simulink library "M160_lib"  (Simulink 7.8)
settings: Solver=FixedStepDiscrete  StartTime=0.0  StopTime=10.0  RelTol=1e-3
PreLoadFcn:
  | update_path
undefined symbols (not defined in the file): Afr_atCool2facLambdaReqCorr_CUR_x, Afr_atCool2facLambdaReqCorr_CUR_y, Afr_atMani2facLambdaReqCorr_CUR_x, Afr_atMani2facLambdaReqCorr_CUR_y, Afr_facLambdaReqMan, Afr_facRatioMan, Afr_facStoich, Afr_flgLambdaReqOverride, Afr_flgRatioOverride, Afr_rpmEngSpdfacRelAir2facLambdaReqBase_MAP_x, Afr_rpmEngSpdfacRelAir2facLambdaReqBase_MAP_y, Afr_rpmEngSpdfacRelAir2facLambdaReqBase_MAP_z, Ais_flgAirInjReacPumpOverride, Ais_stAirInjReacPumpMan, Amc_flgAirMassFlowOverride, Amc_uSens2AirMassFlow_CUR_x, Amc_uSens2AirMassFlow_CUR_y, Amc_uSensMaxValid, Amc_uSensMinValid, Amf_facRelAirMan, Amf_flgAirMassPerStrOverride, Amf_flgRelAirOverride, Amf_flgSwitch2AirMassFlowMeter, Amf_mAirPerStrMan, Amf_pManiEngSpd2facRelAirCorr_MAP_x, Amf_pManiEngSpd2facRelAirCorr_MAP_y, Amf_pManiEngSpd2facRelAirCorr_MAP_z, Amf_rpmEngSpd2facTempCorr_CUR_x, Amf_rpmEngSpd2facTempCorr_CUR_y, Amf_shcSpecGasConst_C, Amf_volEngDisp_C, Apv_facAirPumpRateMan, Apv_factor, Apv_flgAirPumpRateOverride, Apv_tiPeriod_C, Bvc_rVoltDivHigh, Bvc_rVoltDivLow, Bvc_uBattMax, Bvc_uBattMin, CDRV_E_OK_, Cov_facChOverVlvRateMan, Cov_factor, Cov_flgChOverVlvRateOverride, Cov_tiPeriod_C, Cpc_atManiTmp2facPresCorr_CUR_x, Cpc_atManiTmp2facPresCorr_CUR_y, Cpc_flgPChargeOverride, Cpc_uSens2pManiBase_CUR_x, Cpc_uSens2pManiBase_CUR_y, Ctc_rPullUp_C, Ctc_rSens2atCool_CUR_x, Ctc_rSens2atCool_CUR_y, Ctc_uSensMaxValid, Ctc_uSensMinValid, Ctc_uSupply, Doh_OutputDiagnosisOverride, dummy_facAirPumpRateReq, dummy_facChOverVlvRateReq, dummy_flgInterCoolerOverride, dummy_flgKl50Override ... (+243)
libraries: simulink x36, ehooks_lib x3
(part 5 of 8)

== system M160_lib/Actuators/Ivc/Ivc ==
  Opm_idxMode : Inport
  Itc_flgInjCutoff : Inport  Port=2
  Itc_tiInj : Inport  Port=3
  Itc_tiBattDelay : Inport  Port=4
  function : TriggerPort  TriggerType=function-call
  Constant1 : Constant  Value=Ivc_flgInjCutoffOverride
  Constant10 : Constant  Value=Ivc_flgEndOfStartCond
  Constant11 : Constant  Value=Ivc_tiMinThresDeltaEffInjPeriod
  Constant{6,12..15} (5 alike) : Constant  Value=0  OutMin=-72  OutMax=78  OutDataTypeStr=single
  Constant16 : Constant  Value=255  OutDataTypeStr=single
  Constant17 : Constant  Value=0  OutDataTypeStr=single
  Constant18 : Constant  Value=Ivc_tiBattDelayMan
  Constant19 : Constant  Value=Ivc_flgBattDelayOverride
  Constant2 : Constant  Value=Ivc_flgInjCutoff
  Constant20 : Constant  Value=Ivc_degInjAbort
  Constant21 : Constant  Value=Ivc_weea0
  Constant22 : Constant  Value=Ivc_weea1
  Constant23 : Constant  Value=Ivc_weea2
  Constant24 : Constant  Value=Ivc_degOffsetInjEndSimultanInj
  Constant25 : Constant  Value=Ivc_degIntakeClose
  Constant3 : Constant  Value=CDRV_E_OK_
  Constant4 : Constant  Value=Ivc_flgInjTimeOverride
  Constant5 : Constant  Value=Normal
  Constant7 : Constant  Value=Ivc_tiInjMan
  Constant8 : Constant  Value=Ivc_tiInjEff
  Constant9 : Constant  Value=Ivc_flgPostInjCond
  Demux : Demux  Outputs=8
  Demux2 : Demux  Outputs=3
  G1_InjVlvPFI_SetParam : Subsystem  AncestorBlock=ehooks_medc17flex_G1_lib/Library Blocks/INJ/PFI/G1_InjVlvPFI_SetParam  LoadFcn=ehooks_medc17flex_devlib_io_block('load');  InitFcn=ehooks_medc17flex_devlib_io_block('init');  StartFcn=ehooks_medc17flex_devlib_io_block('start');  StopFcn=ehooks_medc17flex_devlib_io_block('stop');  ClipboardFcn=ehooks_medc17flex_devlib_io_block('clipboard', 0); % Second argument just needed to indicate null block. See callback handler.  mask{ChannelName=IGNORED}
      mask prompts: ChannelName "PlaceHolder_IGNORED"
      mask init:
      | ehooks_medc17flex_devlib_io_block('mask_init');
      settings: CopyFcn=ehooks_medc17flex_devlib_io_block('copy');  DeleteFcn=ehooks_medc17flex_devlib_io_block('delete');  UndoDeleteFcn=ehooks_medc17flex_devlib_io_block('undo_delete');  ModelCloseFcn=ehooks_medc17flex_devlib_io_block('model_close');  PreSaveFcn=ehooks_medc17flex_devlib_io_block('pre_save');  PostSaveFcn=ehooks_medc17flex_devlib_io_block('post_save');  NameChangeFcn=ehooks_medc17flex_devlib_io_block('name_change');  DestroyFcn=ehooks_medc17flex_devlib_io_block('destroy', 0); % Second argument just needed to indicate null block. See callback handler.  OpenFcn=ehooks_medc17flex_devlib_io_block('open');  CloseFcn=ehooks_medc17flex_devlib_io_block('close');  ParentCloseFcn=ehooks_medc17flex_devlib_io_block('parent_close');  MoveFcn=ehooks_medc17flex_devlib_io_block('move');
      mask StyleString: popup(IGNORED)
      mask Display: image(imread('InjVlvPfi.jpg'))
  Logical Operator3 : Logic  Operator=OR  AllPortsSameDT=off  OutDataTypeStr=boolean
  Relational Operator : RelationalOperator  Operator=~=  OutDataTypeStr=boolean
  Relational Operator1 : RelationalOperator  Operator=~=  OutDataTypeStr=boolean
  Switch{1..4} (4 alike) : Switch  Threshold=1
  Vector Concatenate : Concatenate  NumInputs=8  Mode=Vector
  Vector Concatenate1 : Concatenate  NumInputs=3  Mode=Vector
  Ivc_flgError : Outport
  wires:
  Switch2/1 -> Vector Concatenate/1, Vector Concatenate/2, Vector Concatenate/3
  Constant15/1 -> Vector Concatenate/8
  Constant14/1 -> Vector Concatenate/7
  Constant13/1 -> Vector Concatenate/6
  Constant12/1 -> Vector Concatenate/5
  Constant6/1 -> Vector Concatenate/4
  Vector Concatenate/1 -> Demux/1  "Ivc_tiInjEffCylInd_Arr"
  Constant8/1 -> G1_InjVlvPFI_SetParam/1(te_i)
  Switch1/1 -> Logical Operator3/2
  Relational Operator/1 -> Logical Operator3/1
  Constant7/1 -> Switch2/1
  Constant4/1 -> Switch2/2
  Itc_tiInj/1 -> Switch2/3
  Constant3/1 -> Relational Operator1/2
  Relational Operator1/1 -> Ivc_flgError/1
  G1_InjVlvPFI_SetParam/1(Cdrv_Error) -> Relational Operator1/1  "Ivc_idxPfiCdrvInterfaceError"
  Constant5/1 -> Relational Operator/2
  Opm_idxMode/1 -> Relational Operator/1
  Itc_flgInjCutoff/1 -> Switch1/3
  Constant2/1 -> Switch1/1
  Constant1/1 -> Switch1/2
  Logical Operator3/1 -> Switch3/2
  Constant16/1 -> Switch3/1
  Constant17/1 -> Switch3/3
  Switch3/1 -> [Ivc_stCutoffPattern_local]  "Ivc_stCutoffPattern"
  Constant18/1 -> Switch4/1
  Constant19/1 -> Switch4/2
  Itc_tiBattDelay/1 -> Switch4/3
  Vector Concatenate1/1 -> Demux2/1  "Ivc_degInjEnd"
  Constant21/1 -> Vector Concatenate1/1
  Constant22/1 -> Vector Concatenate1/2
  Constant23/1 -> Vector Concatenate1/3
  Switch4/1 -> G1_InjVlvPFI_SetParam/11(tvub_w)  "Ivc_tiBattDelay"
  Constant11/1 -> G1_InjVlvPFI_SetParam/10(dtemnkt_w)
  Demux/1 -> G1_InjVlvPFI_SetParam/2(tez_i1)
  Demux/2 -> G1_InjVlvPFI_SetParam/3(tez_i2)
  Demux/3 -> G1_InjVlvPFI_SetParam/4(tez_i3)
  Demux/4 -> G1_InjVlvPFI_SetParam/5(tez_i4)
  Demux/5 -> G1_InjVlvPFI_SetParam/6(tez_i5)
  Demux/6 -> G1_InjVlvPFI_SetParam/7(tez_i6)
  Demux/7 -> G1_InjVlvPFI_SetParam/8(tez_i7)
  Demux/8 -> G1_InjVlvPFI_SetParam/9(tez_i8)
  Constant9/1 -> G1_InjVlvPFI_SetParam/12(B_nsp)
  Constant10/1 -> G1_InjVlvPFI_SetParam/13(B_stendes)
  [Ivc_stCutoffPattern_local] -> G1_InjVlvPFI_SetParam/14(evz_austot)
  Constant20/1 -> G1_InjVlvPFI_SetParam/15(wea)
  Demux2/1 -> G1_InjVlvPFI_SetParam/16(weea_1)
  Demux2/2 -> G1_InjVlvPFI_SetParam/17(weea_2)
  Demux2/3 -> G1_InjVlvPFI_SetParam/18(weea_3)
  Constant24/1 -> G1_InjVlvPFI_SetParam/19(weestim)
  Constant25/1 -> G1_InjVlvPFI_SetParam/20(wes)

== system M160_lib/Actuators/Ivc/Ivc_Diag ==
  function : TriggerPort  TriggerType=function-call
  Constant3 : Constant  Value=CDRV_E_OK_
  Constant8 : Constant  Value=Ivc_flgDiagEntryCondFulfilled
  Constant9 : Constant  Value=Ivc_flgOverrunCutoff
  G1_Inj_Set_DEVE_forPFI : Subsystem  AncestorBlock=ehooks_medc17flex_G1_lib/Library Blocks/INJ/PFI/G1_Inj_Set_DEVE_forPFI  LoadFcn=ehooks_medc17flex_devlib_io_block('load');  InitFcn=ehooks_medc17flex_devlib_io_block('init');  StartFcn=ehooks_medc17flex_devlib_io_block('start');  StopFcn=ehooks_medc17flex_devlib_io_block('stop');  ClipboardFcn=ehooks_medc17flex_devlib_io_block('clipboard', 0); % Second argument just needed to indicate null block. See callback handler.  mask{ChannelName=IGNORED}
      mask prompts: ChannelName "PlaceHolder_IGNORED"
      mask help: InjVlvDeve
      mask init:
      | ehooks_medc17flex_devlib_io_block('mask_init');
      settings: CopyFcn=ehooks_medc17flex_devlib_io_block('copy');  DeleteFcn=ehooks_medc17flex_devlib_io_block('delete');  UndoDeleteFcn=ehooks_medc17flex_devlib_io_block('undo_delete');  ModelCloseFcn=ehooks_medc17flex_devlib_io_block('model_close');  PreSaveFcn=ehooks_medc17flex_devlib_io_block('pre_save');  PostSaveFcn=ehooks_medc17flex_devlib_io_block('post_save');  NameChangeFcn=ehooks_medc17flex_devlib_io_block('name_change');  DestroyFcn=ehooks_medc17flex_devlib_io_block('destroy', 0); % Second argument just needed to indicate null block. See callback handler.  OpenFcn=ehooks_medc17flex_devlib_io_block('open');  CloseFcn=ehooks_medc17flex_devlib_io_block('close');  ParentCloseFcn=ehooks_medc17flex_devlib_io_block('parent_close');  MoveFcn=ehooks_medc17flex_devlib_io_block('move');
      mask StyleString: popup(IGNORED)
      mask Display: image(imread('InjVlvPfi.jpg'))
  Relational Operator1 : RelationalOperator  Operator=~=  OutDataTypeStr=boolean
  Ivc_flgError : Outport
  wires:
  G1_Inj_Set_DEVE_forPFI/1(Cdrv_Error) -> Relational Operator1/1  "Ivc_idxDeveCdrvInterfaceError"
  Relational Operator1/1 -> Ivc_flgError/1
  Constant3/1 -> Relational Operator1/2
  Constant9/1 -> G1_Inj_Set_DEVE_forPFI/2(B_sa)
  Constant8/1 -> G1_Inj_Set_DEVE_forPFI/1(B_desee)

== system M160_lib/Actuators/Ivc/Ivc_Error ==
  Ivc : Inport
  Ivc_Diag : Inport  Port=2
  function : TriggerPort  TriggerType=function-call
  Logical Operator3 : Logic  Operator=OR  AllPortsSameDT=off  OutDataTypeStr=boolean
  Ivc_flgError : Outport
  wires:
  Logical Operator3/1 -> Ivc_flgError/1  "Ivc_flgError"
  Ivc/1 -> Logical Operator3/1
  Ivc_Diag/1 -> Logical Operator3/2

== system M160_lib/Actuators/Mrs/G1_DigOut_Ctrl ==
  state : Inport
  DTC_DigOut_ctrl : DataTypeConversion  OutDataTypeStr=uint8  RndMeth=Nearest
  DTC_Out1 : DataTypeConversion  OutDataTypeStr=boolean
  FlexECU_DevLib_FcnAPI_Wrapper_SFcn : S-Function  FunctionName=ehooks_medc17flex_devlib_basic_io_fcncall  Parameters=NoInputPorts, NoOutputPorts, InputPortDataTypes, OutputPortDataTypes, CFunctionArgTypes, CFunctionName, ChannelName  EnableBusSupport=off  mask{NoInputPorts=1, NoOutputPorts=1, InputPortDataTypes=uint8, OutputPortDataTypes=uint8, CFunctionArgTypes=ret,val, CFunctionName=DevLib_Dio_Set, ChannelName=O_S_MRLY}
      mask prompts: NoInputPorts "Number of input ports"; NoOutputPorts "Number of output ports"; InputPortDataTypes "Input port data types"; OutputPortDataTypes "Output port data types"; CFunctionArgTypes "C function argument types"; CFunctionName "C function name"; ChannelName "Channel (pin) name"
      mask Display: disp('EHOOKS FlexECU\nDevLib Wrapper\nS-Function')
  status : Outport
  wires:
  DTC_DigOut_ctrl/1 -> FlexECU_DevLib_FcnAPI_Wrapper_SFcn/1
  state/1 -> DTC_DigOut_ctrl/1
  FlexECU_DevLib_FcnAPI_Wrapper_SFcn/1 -> DTC_Out1/1
  DTC_Out1/1 -> status/1

== system M160_lib/Actuators/Mrs/G1_DigOut_GetError ==
  DTC_DigOut_GetError : DataTypeConversion  OutDataTypeStr=single
  FlexECU_DevLib_FcnAPI_Wrapper_SFcn : S-Function  FunctionName=ehooks_medc17flex_devlib_basic_io_fcncall  Parameters=NoInputPorts, NoOutputPorts, InputPortDataTypes, OutputPortDataTypes, CFunctionArgTypes, CFunctionName, ChannelName  EnableBusSupport=off  mask{NoInputPorts=0, NoOutputPorts=1, InputPortDataTypes=, OutputPortDataTypes=uint8, CFunctionArgTypes=ret, CFunctionName=DevLib_DioSet_GetError, ChannelName=O_S_MRLY}
      mask prompts: NoInputPorts "Number of input ports"; NoOutputPorts "Number of output ports"; InputPortDataTypes "Input port data types"; OutputPortDataTypes "Output port data types"; CFunctionArgTypes "C function argument types"; CFunctionName "C function name"; ChannelName "Channel (pin) name"
      mask Display: disp('EHOOKS FlexECU\nDevLib Wrapper\nS-Function')
  status : Outport
  wires:
  DTC_DigOut_GetError/1 -> status/1
  FlexECU_DevLib_FcnAPI_Wrapper_SFcn/1 -> DTC_DigOut_GetError/1

== system M160_lib/Actuators/Str/G1_DigOut_Ctrl ==
  state : Inport
  DTC_DigOut_ctrl : DataTypeConversion  OutDataTypeStr=uint8  RndMeth=Nearest
  DTC_Out1 : DataTypeConversion  OutDataTypeStr=boolean
  FlexECU_DevLib_FcnAPI_Wrapper_SFcn : S-Function  FunctionName=ehooks_medc17flex_devlib_basic_io_fcncall  Parameters=NoInputPorts, NoOutputPorts, InputPortDataTypes, OutputPortDataTypes, CFunctionArgTypes, CFunctionName, ChannelName  EnableBusSupport=off  mask{NoInputPorts=1, NoOutputPorts=1, InputPortDataTypes=uint8, OutputPortDataTypes=uint8, CFunctionArgTypes=ret,val, CFunctionName=DevLib_Dio_Set, ChannelName=O_S_RL34}
      mask prompts: NoInputPorts "Number of input ports"; NoOutputPorts "Number of output ports"; InputPortDataTypes "Input port data types"; OutputPortDataTypes "Output port data types"; CFunctionArgTypes "C function argument types"; CFunctionName "C function name"; ChannelName "Channel (pin) name"
      mask Display: disp('EHOOKS FlexECU\nDevLib Wrapper\nS-Function')
  status : Outport
  wires:
  DTC_DigOut_ctrl/1 -> FlexECU_DevLib_FcnAPI_Wrapper_SFcn/1
  state/1 -> DTC_DigOut_ctrl/1
  FlexECU_DevLib_FcnAPI_Wrapper_SFcn/1 -> DTC_Out1/1
  DTC_Out1/1 -> status/1

== system M160_lib/Actuators/Str/G1_DigOut_GetError ==
  DTC_DigOut_GetError : DataTypeConversion  OutDataTypeStr=single
  FlexECU_DevLib_FcnAPI_Wrapper_SFcn : S-Function  FunctionName=ehooks_medc17flex_devlib_basic_io_fcncall  Parameters=NoInputPorts, NoOutputPorts, InputPortDataTypes, OutputPortDataTypes, CFunctionArgTypes, CFunctionName, ChannelName  EnableBusSupport=off  mask{NoInputPorts=0, NoOutputPorts=1, InputPortDataTypes=, OutputPortDataTypes=uint8, CFunctionArgTypes=ret, CFunctionName=DevLib_DioSet_GetError, ChannelName=O_S_RL34}
      mask prompts: NoInputPorts "Number of input ports"; NoOutputPorts "Number of output ports"; InputPortDataTypes "Input port data types"; OutputPortDataTypes "Output port data types"; CFunctionArgTypes "C function argument types"; CFunctionName "C function name"; ChannelName "Channel (pin) name"
      mask Display: disp('EHOOKS FlexECU\nDevLib Wrapper\nS-Function')
  status : Outport
  wires:
  DTC_DigOut_GetError/1 -> status/1
  FlexECU_DevLib_FcnAPI_Wrapper_SFcn/1 -> DTC_DigOut_GetError/1

== system M160_lib/Actuators/Tvc/Limiter ==
  max : Inport
  in : Inport  Port=2
  min : Inport  Port=3
  Saturation Dynamic : simulink/Discontinuities/Saturation Dynamic  OutMin=[]  OutMax=[]  OutDataTypeStr=Inherit: Same as second input  OutDataType=fixdt(1, 16)  OutScaling=2^-10  DoSatur=off
  return : Outport
  wires:
  max/1 -> Saturation Dynamic/1
  in/1 -> Saturation Dynamic/2
  min/1 -> Saturation Dynamic/3
  Saturation Dynamic/1 -> return/1

== system M160_lib/Actuators/Tvc/ThrottleValveControl ==
  Tvc_flgPosError : Inport
  Tvc_facThrValve : Inport  Port=2
  Tvc_facThrValveReq : Inport  Port=3
  Add : Sum  OutDataTypeStr=Inherit: Same as first input
  Constan1 : Constant  Value=0.0  OutDataTypeStr=single
  Constan2 : Constant  Value=0.01  OutDataTypeStr=single
  Constant1 : Constant  Value=Tvc_facDutycyclePilotControlPos  OutDataTypeStr=single
  Constant2 : Constant  Value=Tvc_facDutycyclePilotControlNeg  OutDataTypeStr=single
  Constant3 : Constant  Value=Tvc_flgThrValveDutycycleOverride
  Constant4 : Constant  Value=Tvc_facThrValveDutycycleMan
  Constant5 : Constant  Value=Tvc_tiTnDutycycle
  Constant6 : Constant  Value=Tvc_tiTvDutycycle
  Constant7 : Constant  Value=Tvc_facKDutycycle
  Constant8 : Constant  Value=Tvc_facDutycyclePIDLimitMax
  Constant9 : Constant  Value=Tvc_facDutycyclePIDLimitMin
  Logical Operator1 : Logic  Operator=NOT  AllPortsSameDT=off  OutDataTypeStr=boolean
  Manual Switch : simulink/Signal Routing/Manual Switch  sw=1  action=0  varsize=off
  PID_Limit_AWU : Subsystem
      mask Description: PID_Limit_AWU
      mask Display: image(imread('PID_Limit_AWU.jpg'))
  PID_Limit_AWU_Fcn : Subsystem
      mask Description: PID_Limit_AWU_Fcn
      mask Display: image(imread('PID_Limit_AWU.jpg'))
  Relational Operator : RelationalOperator  Operator=<  OutDataTypeStr=boolean
  Subtract : Sum  Inputs=+-  OutDataTypeStr=Inherit: Same as first input
  Switch : Switch  Threshold=1
  Switch1 : Switch  Threshold=1
  Tvc_facDutycycle : Outport
  wires:
  Constant3/1 -> Switch1/2
  Constant4/1 -> Switch1/1
  Add/1 -> Switch1/3
  Constan1/1 -> Relational Operator/2
  Relational Operator/1 -> Switch/2
  Switch/1 -> Add/1
  Switch1/1 -> Tvc_facDutycycle/1
  Tvc_flgPosError/1 -> Logical Operator1/1
  Constant5/1 -> PID_Limit_AWU/1(Tn)
  Constan2/1 -> PID_Limit_AWU/3(Ta)
  Subtract/1 -> PID_Limit_AWU/5(in), PID_Limit_AWU_Fcn/1(in)
  Constant6/1 -> PID_Limit_AWU/2(Tv)
  Constant7/1 -> PID_Limit_AWU/4(Kp)
  Tvc_facThrValveReq/1 -> Subtract/2
  Tvc_facThrValve/1 -> Subtract/1, Relational Operator/1
  Constant2/1 -> Switch/1
  Constant1/1 -> Switch/3
  Logical Operator1/1 -> PID_Limit_AWU/6(initValue), PID_Limit_AWU_Fcn/2(initValue)
  Constant8/1 -> PID_Limit_AWU/7(outMax)
  Constant9/1 -> PID_Limit_AWU/8(outMin)
  PID_Limit_AWU_Fcn/1(Tvc_facDutycycleCorr) -> Manual Switch/2  "Tvc_facDutycycleCorr_Fcn"
  PID_Limit_AWU/1(Tvc_facDutycycleCorr) -> Manual Switch/1  "Tvc_facDutycycleCorr"
  Manual Switch/1 -> Add/2

== system M160_lib/Actuators/Tvc/ThrottleValveOutput ==
  Tvc_flgPosError : Inport
  Tvc_facDutycycle : Inport  Port=2
  Constant1 : Constant  Value=Tvc_tiPeriod_C
  Constant3 : Constant  Value=Lo_
  Constant5 : Constant  Value=Normal
  G1_HbridgeOut_Ctrl : Subsystem  AncestorBlock=ehooks_medc17flex_G1_lib/Library Blocks/Basic_IO/Outputs/G1_HbridgeOut_Ctrl  LoadFcn=ehooks_medc17flex_devlib_io_block('load');  InitFcn=ehooks_medc17flex_devlib_io_block('init');  StartFcn=ehooks_medc17flex_devlib_io_block('start');  StopFcn=ehooks_medc17flex_devlib_io_block('stop');  ClipboardFcn=ehooks_medc17flex_devlib_io_block('clipboard', 0); % Second argument just needed to indicate null block. See callback handler.  mask{ChannelName=O_T_DC1}
      mask prompts: ChannelName "Channel name"
      mask init:
      | ehooks_medc17flex_devlib_io_block('mask_init');
      settings: AttributesFormatString=Channel name: '%<ChannelName>'  CopyFcn=ehooks_medc17flex_devlib_io_block('copy');  DeleteFcn=ehooks_medc17flex_devlib_io_block('delete');  UndoDeleteFcn=ehooks_medc17flex_devlib_io_block('undo_delete');  ModelCloseFcn=ehooks_medc17flex_devlib_io_block('model_close');  PreSaveFcn=ehooks_medc17flex_devlib_io_block('pre_save');  PostSaveFcn=ehooks_medc17flex_devlib_io_block('post_save');  NameChangeFcn=ehooks_medc17flex_devlib_io_block('name_change');  DestroyFcn=ehooks_medc17flex_devlib_io_block('destroy', 0); % Second argument just needed to indicate null block. See callback handler.  OpenFcn=ehooks_medc17flex_devlib_io_block('open');  CloseFcn=ehooks_medc17flex_devlib_io_block('close');  ParentCloseFcn=ehooks_medc17flex_devlib_io_block('parent_close');  MoveFcn=ehooks_medc17flex_devlib_io_block('move');
      mask StyleString: popup(<empty>|O_T_DC1|O_T_DC2|O_T_DC3)
      mask Display: image(imread('Output_HBridge.jpg'))
  G1_Hbridge_Get_error : Subsystem  AncestorBlock=ehooks_medc17flex_G1_lib/Library Blocks/Basic_IO/Outputs/G1_Hbridge_Get_error  LoadFcn=ehooks_medc17flex_devlib_io_block('load');  InitFcn=ehooks_medc17flex_devlib_io_block('init');  StartFcn=ehooks_medc17flex_devlib_io_block('start');  StopFcn=ehooks_medc17flex_devlib_io_block('stop');  ClipboardFcn=ehooks_medc17flex_devlib_io_block('clipboard', 0); % Second argument just needed to indicate null block. See callback handler.  mask{ChannelName=O_T_DC1}
      mask prompts: ChannelName "Channel name"
      mask init:
      | ehooks_medc17flex_devlib_io_block('mask_init');
      settings: AttributesFormatString=Channel name: '%<ChannelName>'  CopyFcn=ehooks_medc17flex_devlib_io_block('copy');  DeleteFcn=ehooks_medc17flex_devlib_io_block('delete');  UndoDeleteFcn=ehooks_medc17flex_devlib_io_block('undo_delete');  ModelCloseFcn=ehooks_medc17flex_devlib_io_block('model_close');  PreSaveFcn=ehooks_medc17flex_devlib_io_block('pre_save');  PostSaveFcn=ehooks_medc17flex_devlib_io_block('post_save');  NameChangeFcn=ehooks_medc17flex_devlib_io_block('name_change');  DestroyFcn=ehooks_medc17flex_devlib_io_block('destroy', 0); % Second argument just needed to indicate null block. See callback handler.  OpenFcn=ehooks_medc17flex_devlib_io_block('open');  CloseFcn=ehooks_medc17flex_devlib_io_block('close');  ParentCloseFcn=ehooks_medc17flex_devlib_io_block('parent_close');  MoveFcn=ehooks_medc17flex_devlib_io_block('move');
      mask StyleString: popup(<empty>|O_T_DC1|O_T_DC2|O_T_DC3)
      mask Display: image(imread('Output_HBridge_Diagnosis.jpg'))
  Interval Test : simulink/Logic and Bit Operations/Interval Test  IntervalClosedRight=on  uplimit=1  IntervalClosedLeft=on  lowlimit=-1  OutDataTypeStr=boolean
  Logical Operator : Logic  Operator=OR  Inputs=3  AllPortsSameDT=off  OutDataTypeStr=boolean
  Relational Operator : RelationalOperator  Operator=~=  OutDataTypeStr=boolean
  Tvc_stHBridge : Outport
  Tvc_stDiagnosis : Outport  Port=2
  wires:
  Constant1/1 -> G1_HbridgeOut_Ctrl/3(period)
  Tvc_facDutycycle/1 -> G1_HbridgeOut_Ctrl/1(dutycycle), Interval Test/1
  G1_HbridgeOut_Ctrl/1(status) -> Tvc_stHBridge/1
  Logical Operator/1 -> G1_HbridgeOut_Ctrl/2(disable)
  Interval Test/1 -> Logical Operator/1
  Constant3/1 -> G1_HbridgeOut_Ctrl/4(level)
  G1_Hbridge_Get_error/1(status) -> Tvc_stDiagnosis/1
  [Opm_idxMode_global] -> Relational Operator/1
  Constant5/1 -> Relational Operator/2
  Tvc_flgPosError/1 -> Logical Operator/2
  Relational Operator/1 -> Logical Operator/3

== system M160_lib/Actuators/Tvc/ThrottleValvePosition ==
  Abs : Abs
  Add : Sum  OutDataTypeStr=Inherit: Same as first input
  Constan1 : Constant  Value=0.05  OutDataTypeStr=single
  Constant : Constant  Value=2  OutDataTypeStr=single
  Divide : Product  Inputs=*/  OutDataTypeStr=Inherit: Same as first input
  G1_ADC_Input_Receive : Subsystem  AncestorBlock=ehooks_medc17flex_G1_lib/Library Blocks/Basic_IO/Inputs/G1_ADC_Input_Receive  LoadFcn=ehooks_medc17flex_devlib_io_block('load');  InitFcn=ehooks_medc17flex_devlib_io_block('init');  StartFcn=ehooks_medc17flex_devlib_io_block('start');  StopFcn=ehooks_medc17flex_devlib_io_block('stop');  ClipboardFcn=ehooks_medc17flex_devlib_io_block('clipboard', 0); % Second argument just needed to indicate null block. See callback handler.  mask{ChannelName=I_A_AN01}
      mask prompts: ChannelName "Channel name"
      mask init:
      | ehooks_medc17flex_devlib_io_block('mask_init');
      settings: AttributesFormatString=Channel name: '%<ChannelName>'  CopyFcn=ehooks_medc17flex_devlib_io_block('copy');  DeleteFcn=ehooks_medc17flex_devlib_io_block('delete');  UndoDeleteFcn=ehooks_medc17flex_devlib_io_block('undo_delete');  ModelCloseFcn=ehooks_medc17flex_devlib_io_block('model_close');  PreSaveFcn=ehooks_medc17flex_devlib_io_block('pre_save');  PostSaveFcn=ehooks_medc17flex_devlib_io_block('post_save');  NameChangeFcn=ehooks_medc17flex_devlib_io_block('name_change');  DestroyFcn=ehooks_medc17flex_devlib_io_block('destroy', 0); % Second argument just needed to indicate null block. See callback handler.  OpenFcn=ehooks_medc17flex_devlib_io_block('open');  CloseFcn=ehooks_medc17flex_devlib_io_block('close');  ParentCloseFcn=ehooks_medc17flex_devlib_io_block('parent_close');  MoveFcn=ehooks_medc17flex_devlib_io_block('move');
      mask StyleString: popup(<empty>|I_A_AN01|I_A_AN02|I_A_AN03|I_A_AN05|I_A_AN06|I_A_AN07|I_A_AN08|I_A_AN10|I_A_AN11|I_A_AN12|I_A_AN13|I_A_AN14|I_A_AN15|I_A_AN16|I_A_AN17|I_A_AN18|I_A_AN19|I_A_AN20|I_A_AN21|I_A_AN23|I_A_AN32|I_A_AN35|I_A_AN36|I_A_AN37|I_A_AN39|I_A_AN100|I_A_AN101|I_A_AN103|I_A_AN104|I_A_AN105|I_A_AN106)
      mask Display: image(imread('Input_Analog.jpg'))
  G1_ADC_Input_Receive1 : Subsystem  AncestorBlock=ehooks_medc17flex_G1_lib/Library Blocks/Basic_IO/Inputs/G1_ADC_Input_Receive  LoadFcn=ehooks_medc17flex_devlib_io_block('load');  InitFcn=ehooks_medc17flex_devlib_io_block('init');  StartFcn=ehooks_medc17flex_devlib_io_block('start');  StopFcn=ehooks_medc17flex_devlib_io_block('stop');  ClipboardFcn=ehooks_medc17flex_devlib_io_block('clipboard', 0); % Second argument just needed to indicate null block. See callback handler.  mask{ChannelName=I_A_AN02}
      mask prompts: ChannelName "Channel name"
      mask init:
      | ehooks_medc17flex_devlib_io_block('mask_init');
      settings: AttributesFormatString=Channel name: '%<ChannelName>'  CopyFcn=ehooks_medc17flex_devlib_io_block('copy');  DeleteFcn=ehooks_medc17flex_devlib_io_block('delete');  UndoDeleteFcn=ehooks_medc17flex_devlib_io_block('undo_delete');  ModelCloseFcn=ehooks_medc17flex_devlib_io_block('model_close');  PreSaveFcn=ehooks_medc17flex_devlib_io_block('pre_save');  PostSaveFcn=ehooks_medc17flex_devlib_io_block('post_save');  NameChangeFcn=ehooks_medc17flex_devlib_io_block('name_change');  DestroyFcn=ehooks_medc17flex_devlib_io_block('destroy', 0); % Second argument just needed to indicate null block. See callback handler.  OpenFcn=ehooks_medc17flex_devlib_io_block('open');  CloseFcn=ehooks_medc17flex_devlib_io_block('close');  ParentCloseFcn=ehooks_medc17flex_devlib_io_block('parent_close');  MoveFcn=ehooks_medc17flex_devlib_io_block('move');
      mask StyleString: popup(<empty>|I_A_AN01|I_A_AN02|I_A_AN03|I_A_AN05|I_A_AN06|I_A_AN07|I_A_AN08|I_A_AN10|I_A_AN11|I_A_AN12|I_A_AN13|I_A_AN14|I_A_AN15|I_A_AN16|I_A_AN17|I_A_AN18|I_A_AN19|I_A_AN20|I_A_AN21|I_A_AN23|I_A_AN32|I_A_AN35|I_A_AN36|I_A_AN37|I_A_AN39|I_A_AN100|I_A_AN101|I_A_AN103|I_A_AN104|I_A_AN105|I_A_AN106)
      mask Display: image(imread('Input_Analog.jpg'))
  Interval Test : simulink/Logic and Bit Operations/Interval Test  IntervalClosedRight=on  uplimit=Tvc_uSensMaxValid  IntervalClosedLeft=on  lowlimit=Tvc_uSensMinValid  OutDataTypeStr=boolean
  Interval Test1 : simulink/Logic and Bit Operations/Interval Test  IntervalClosedRight=on  uplimit=Tvc_uSensMaxValid  IntervalClosedLeft=on  lowlimit=Tvc_uSensMinValid  OutDataTypeStr=boolean
  Logical Operator{,1..3} (4 alike) : Logic  Operator=NOT  AllPortsSameDT=off  OutDataTypeStr=boolean
  Logical Operator4 : Logic  Operator=OR  Inputs=5  AllPortsSameDT=off  OutDataTypeStr=boolean
  Relational Oprator : RelationalOperator  Operator=>  OutDataTypeStr=boolean
  Subtract : Sum  Inputs=+-  OutDataTypeStr=Inherit: Same as first input
  Tvc_uSens2facThrValve1_CUR : Lookup_n-D  NumberOfTableDimensions=1  BreakpointsForDimension1=Tvc_uSens2facThrValve1_CUR_x  Table=Tvc_uSens2facThrValve1_CUR_y  ExtrapMethod=Clip  OutDataTypeStr=Inherit: Inherit from 'Table data'  InputSameDT=on
  Tvc_uSens2facThrValve2_CUR : Lookup_n-D  NumberOfTableDimensions=1  BreakpointsForDimension1=Tvc_uSens2facThrValve2_CUR_x  Table=Tvc_uSens2facThrValve2_CUR_y  ExtrapMethod=Clip  OutDataTypeStr=Inherit: Inherit from 'Table data'  InputSameDT=on
  Tvc_flgPosError : Outport
  Tvc_facThrValve : Outport  Port=2
  wires:
  G1_ADC_Input_Receive/1(status) -> Logical Operator/1  "Tvc_stIO1"
  G1_ADC_Input_Receive/2(uRaw) -> Tvc_uSens2facThrValve1_CUR/1, Interval Test/1  "Tvc_uSens1"
  G1_ADC_Input_Receive1/1(status) -> Logical Operator2/1  "Tvc_stIO2"
  G1_ADC_Input_Receive1/2(uRaw) -> Tvc_uSens2facThrValve2_CUR/1, Interval Test1/1  "Tvc_uSens2"
  Interval Test/1 -> Logical Operator1/1
  Interval Test1/1 -> Logical Operator3/1
  Tvc_uSens2facThrValve1_CUR/1 -> Add/1, Subtract/1  "Tvc_facThrValve1"
  Tvc_uSens2facThrValve2_CUR/1 -> Add/2, Subtract/2  "Tvc_facThrValve2"
  Add/1 -> Divide/1
  Constant/1 -> Divide/2
  Subtract/1 -> Abs/1
  Abs/1 -> Relational Oprator/1
  Constan1/1 -> Relational Oprator/2
  Logical Operator4/1 -> Tvc_flgPosError/1
  Logical Operator/1 -> Logical Operator4/1
  Logical Operator1/1 -> Logical Operator4/2
  Logical Operator2/1 -> Logical Operator4/3
  Logical Operator3/1 -> Logical Operator4/4
  Relational Oprator/1 -> Logical Operator4/5
  Divide/1 -> Tvc_facThrValve/1

== system M160_lib/Actuators/Wcs/G1_DigOut_Ctrl ==
  state : Inport
  DTC_DigOut_ctrl : DataTypeConversion  OutDataTypeStr=uint8  RndMeth=Nearest
  DTC_Out1 : DataTypeConversion  OutDataTypeStr=boolean
  FlexECU_DevLib_FcnAPI_Wrapper_SFcn : S-Function  FunctionName=ehooks_medc17flex_devlib_basic_io_fcncall  Parameters=NoInputPorts, NoOutputPorts, InputPortDataTypes, OutputPortDataTypes, CFunctionArgTypes, CFunctionName, ChannelName  EnableBusSupport=off  mask{NoInputPorts=1, NoOutputPorts=1, InputPortDataTypes=uint8, OutputPortDataTypes=uint8, CFunctionArgTypes=ret,val, CFunctionName=DevLib_Dio_Set, ChannelName=O_S_RL14}
      mask prompts: NoInputPorts "Number of input ports"; NoOutputPorts "Number of output ports"; InputPortDataTypes "Input port data types"; OutputPortDataTypes "Output port data types"; CFunctionArgTypes "C function argument types"; CFunctionName "C function name"; ChannelName "Channel (pin) name"
      mask Display: disp('EHOOKS FlexECU\nDevLib Wrapper\nS-Function')
  status : Outport
  wires:
  DTC_DigOut_ctrl/1 -> FlexECU_DevLib_FcnAPI_Wrapper_SFcn/1
  state/1 -> DTC_DigOut_ctrl/1
  FlexECU_DevLib_FcnAPI_Wrapper_SFcn/1 -> DTC_Out1/1
  DTC_Out1/1 -> status/1

== system M160_lib/Actuators/Wcs/G1_DigOut_GetError ==
  DTC_DigOut_GetError : DataTypeConversion  OutDataTypeStr=single
  FlexECU_DevLib_FcnAPI_Wrapper_SFcn : S-Function  FunctionName=ehooks_medc17flex_devlib_basic_io_fcncall  Parameters=NoInputPorts, NoOutputPorts, InputPortDataTypes, OutputPortDataTypes, CFunctionArgTypes, CFunctionName, ChannelName  EnableBusSupport=off  mask{NoInputPorts=0, NoOutputPorts=1, InputPortDataTypes=, OutputPortDataTypes=uint8, CFunctionArgTypes=ret, CFunctionName=DevLib_DioSet_GetError, ChannelName=O_S_RL14}
      mask prompts: NoInputPorts "Number of input ports"; NoOutputPorts "Number of output ports"; InputPortDataTypes "Input port data types"; OutputPortDataTypes "Output port data types"; CFunctionArgTypes "C function argument types"; CFunctionName "C function name"; ChannelName "Channel (pin) name"
      mask Display: disp('EHOOKS FlexECU\nDevLib Wrapper\nS-Function')
  status : Outport
  wires:
  DTC_DigOut_GetError/1 -> status/1
  FlexECU_DevLib_FcnAPI_Wrapper_SFcn/1 -> DTC_DigOut_GetError/1

== system M160_lib/Actuators/Wcs/Hysteresis_Delta_RSP ==
  in : Inport
  Relay : Relay  OnSwitchValue=Wcs_atCoolantMax  OffSwitchValue=Wcs_atCoolantMax-Wcs_atCoolantHyst  OutDataTypeStr=Inherit: Inherit via back propagation
  return : Outport
  wires:
  in/1 -> Relay/1
  Relay/1 -> return/1

== system M160_lib/Actuators/Wgc/G1_PWM_Output_Ctrl ==
  dutycycle : Inport
  period : Inport  Port=2
  factor : Inport  Port=3
  level : Inport  Port=4
  DTC_PwmOut_DutyCycle : DataTypeConversion  OutDataTypeStr=int16  RndMeth=Nearest
  DTC_PwmOut_ErrorInfo : DataTypeConversion  OutDataTypeStr=boolean
  DTC_PwmOut_Level : DataTypeConversion  OutDataTypeStr=int16  RndMeth=Nearest
  DTC_PwmOut_Period : DataTypeConversion  OutDataTypeStr=int16  RndMeth=Nearest
  DTC_PwmOut_Period1 : DataTypeConversion  OutDataTypeStr=uint8  RndMeth=Nearest
  FlexECU_DevLib_FcnAPI_Wrapper_SFcn : S-Function  FunctionName=ehooks_medc17flex_devlib_basic_io_fcncall  Parameters=NoInputPorts, NoOutputPorts, InputPortDataTypes, OutputPortDataTypes, CFunctionArgTypes, CFunctionName, ChannelName  EnableBusSupport=off  mask{NoInputPorts=4, NoOutputPorts=1, InputPortDataTypes=int16,int16, int16, uint8, OutputPortDataTypes=uint8, CFunctionArgTypes=ret,val,val,val,val, CFunctionName=DevLib_Pwm_Out, ChannelName=O_T_RL22}
      mask prompts: NoInputPorts "Number of input ports"; NoOutputPorts "Number of output ports"; InputPortDataTypes "Input port data types"; OutputPortDataTypes "Output port data types"; CFunctionArgTypes "C function argument types"; CFunctionName "C function name"; ChannelName "Channel (pin) name"
      mask Display: disp('EHOOKS FlexECU\nDevLib Wrapper\nS-Function')
  Gain : Gain  Gain=100
  status : Outport
  wires:
  Gain/1 -> DTC_PwmOut_DutyCycle/1
  dutycycle/1 -> Gain/1
  level/1 -> DTC_PwmOut_Period1/1
  DTC_PwmOut_Period1/1 -> FlexECU_DevLib_FcnAPI_Wrapper_SFcn/4
  FlexECU_DevLib_FcnAPI_Wrapper_SFcn/1 -> DTC_PwmOut_ErrorInfo/1
  period/1 -> DTC_PwmOut_Period/1
  factor/1 -> DTC_PwmOut_Level/1
  DTC_PwmOut_DutyCycle/1 -> FlexECU_DevLib_FcnAPI_Wrapper_SFcn/1
  DTC_PwmOut_Period/1 -> FlexECU_DevLib_FcnAPI_Wrapper_SFcn/2
  DTC_PwmOut_Level/1 -> FlexECU_DevLib_FcnAPI_Wrapper_SFcn/3
  DTC_PwmOut_ErrorInfo/1 -> status/1

== system M160_lib/Actuators/Wgc/G1_PwmOut_Get_error ==
  DTC_PwmOut_GetError : DataTypeConversion  OutDataTypeStr=single
  FlexECU_DevLib_FcnAPI_Wrapper_SFcn : S-Function  FunctionName=ehooks_medc17flex_devlib_basic_io_fcncall  Parameters=NoInputPorts, NoOutputPorts, InputPortDataTypes, OutputPortDataTypes, CFunctionArgTypes, CFunctionName, ChannelName  EnableBusSupport=off  mask{NoInputPorts=0, NoOutputPorts=1, InputPortDataTypes=, OutputPortDataTypes=uint8, CFunctionArgTypes=ret, CFunctionName=DevLib_PwmOut_GetError, ChannelName=O_T_RL22}
      mask prompts: NoInputPorts "Number of input ports"; NoOutputPorts "Number of output ports"; InputPortDataTypes "Input port data types"; OutputPortDataTypes "Output port data types"; CFunctionArgTypes "C function argument types"; CFunctionName "C function name"; ChannelName "Channel (pin) name"
      mask Display: disp('EHOOKS FlexECU\nDevLib Wrapper\nS-Function')
  status : Outport
  wires:
  DTC_PwmOut_GetError/1 -> status/1
  FlexECU_DevLib_FcnAPI_Wrapper_SFcn/1 -> DTC_PwmOut_GetError/1

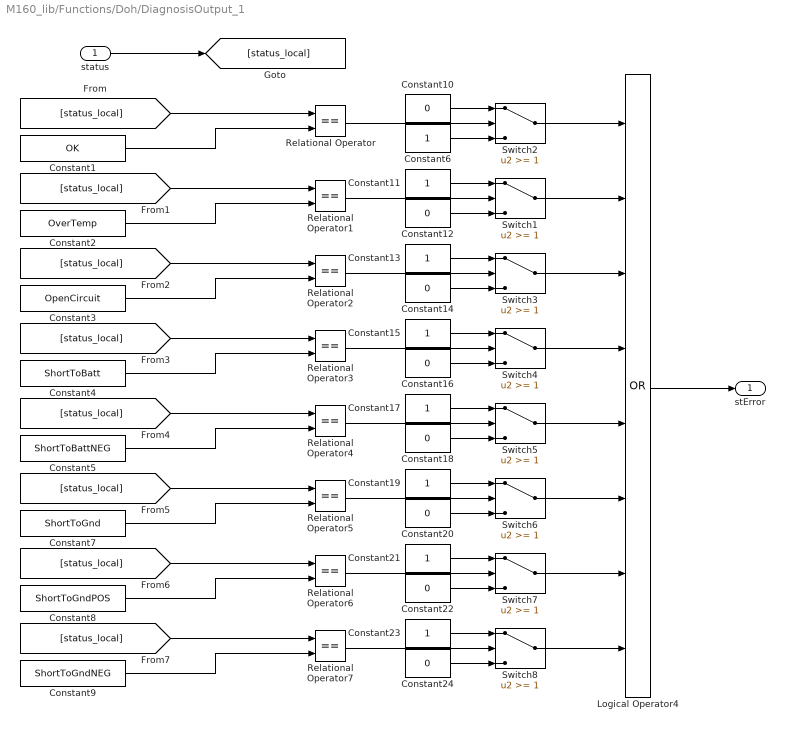
== system M160_lib/Functions/Doh/DiagnosisOutput_1 ==
  status : Inport
  Constant1 : Constant  Value=OK
  Constant{10,12,14,16,18,20,22,24} (8 alike) : Constant  Value=0  OutDataTypeStr=boolean
  Constant{6,11,13,15,17,19,21,23} (8 alike) : Constant  OutDataTypeStr=boolean
  Constant2 : Constant  Value=OverTemp
  Constant3 : Constant  Value=OpenCircuit
  Constant4 : Constant  Value=ShortToBatt
  Constant5 : Constant  Value=ShortToBattNEG
  Constant7 : Constant  Value=ShortToGnd
  Constant8 : Constant  Value=ShortToGndPOS
  Constant9 : Constant  Value=ShortToGndNEG
  Logical Operator4 : Logic  Operator=OR  Inputs=8  AllPortsSameDT=off  OutDataTypeStr=boolean
  Relational Operator{,1..7} (8 alike) : RelationalOperator  Operator===  OutDataTypeStr=boolean
  Switch{1..8} (8 alike) : Switch  Threshold=1
  stError : Outport
  wires:
  Constant1/1 -> Relational Operator/2
  status/1 -> [status_local]
  [status_local] -> Relational Operator/1
  Constant2/1 -> Relational Operator1/2
  [status_local] -> Relational Operator1/1
  Constant3/1 -> Relational Operator2/2
  [status_local] -> Relational Operator2/1
  Constant4/1 -> Relational Operator3/2
  [status_local] -> Relational Operator3/1
  Constant5/1 -> Relational Operator4/2
  [status_local] -> Relational Operator4/1
  Constant7/1 -> Relational Operator5/2
  [status_local] -> Relational Operator5/1
  Constant8/1 -> Relational Operator6/2
  [status_local] -> Relational Operator6/1
  Constant9/1 -> Relational Operator7/2
  [status_local] -> Relational Operator7/1
  Relational Operator/1 -> Switch2/2
  Constant6/1 -> Switch2/3
  Logical Operator4/1 -> stError/1
  Constant10/1 -> Switch2/1
  Constant12/1 -> Switch1/3
  Constant11/1 -> Switch1/1
  Relational Operator1/1 -> Switch1/2
  Constant14/1 -> Switch3/3
  Constant13/1 -> Switch3/1
  Relational Operator2/1 -> Switch3/2
  Constant16/1 -> Switch4/3
  Constant15/1 -> Switch4/1
  Relational Operator3/1 -> Switch4/2
  Constant18/1 -> Switch5/3
  Constant17/1 -> Switch5/1
  Relational Operator4/1 -> Switch5/2
  Constant20/1 -> Switch6/3
  Constant19/1 -> Switch6/1
  Relational Operator5/1 -> Switch6/2
  Constant22/1 -> Switch7/3
  Constant21/1 -> Switch7/1
  Relational Operator6/1 -> Switch7/2
  Constant24/1 -> Switch8/3
  Constant23/1 -> Switch8/1
  Relational Operator7/1 -> Switch8/2
  Switch2/1 -> Logical Operator4/1
  Switch1/1 -> Logical Operator4/2
  Switch3/1 -> Logical Operator4/3
  Switch4/1 -> Logical Operator4/4
  Switch5/1 -> Logical Operator4/5
  Switch6/1 -> Logical Operator4/6
  Switch7/1 -> Logical Operator4/7
  Switch8/1 -> Logical Operator4/8

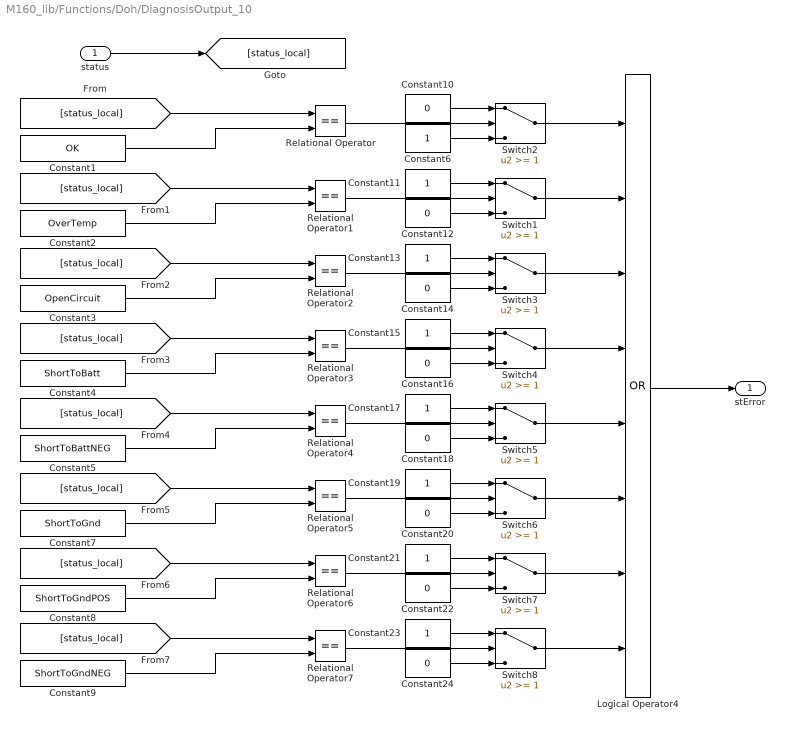
== system M160_lib/Functions/Doh/DiagnosisOutput_10 ==
  status : Inport
  Constant1 : Constant  Value=OK
  Constant{10,12,14,16,18,20,22,24} (8 alike) : Constant  Value=0  OutDataTypeStr=boolean
  Constant{6,11,13,15,17,19,21,23} (8 alike) : Constant  OutDataTypeStr=boolean
  Constant2 : Constant  Value=OverTemp
  Constant3 : Constant  Value=OpenCircuit
  Constant4 : Constant  Value=ShortToBatt
  Constant5 : Constant  Value=ShortToBattNEG
  Constant7 : Constant  Value=ShortToGnd
  Constant8 : Constant  Value=ShortToGndPOS
  Constant9 : Constant  Value=ShortToGndNEG
  Logical Operator4 : Logic  Operator=OR  Inputs=8  AllPortsSameDT=off  OutDataTypeStr=boolean
  Relational Operator{,1..7} (8 alike) : RelationalOperator  Operator===  OutDataTypeStr=boolean
  Switch{1..8} (8 alike) : Switch  Threshold=1
  stError : Outport
  wires:
  Switch8/1 -> Logical Operator4/8
  Switch7/1 -> Logical Operator4/7
  Switch6/1 -> Logical Operator4/6
  Switch5/1 -> Logical Operator4/5
  Switch4/1 -> Logical Operator4/4
  Switch3/1 -> Logical Operator4/3
  Switch1/1 -> Logical Operator4/2
  Switch2/1 -> Logical Operator4/1
  Relational Operator7/1 -> Switch8/2
  Constant23/1 -> Switch8/1
  Constant24/1 -> Switch8/3
  Relational Operator6/1 -> Switch7/2
  Constant21/1 -> Switch7/1
  Constant22/1 -> Switch7/3
  Relational Operator5/1 -> Switch6/2
  Constant19/1 -> Switch6/1
  Constant20/1 -> Switch6/3
  Relational Operator4/1 -> Switch5/2
  Constant17/1 -> Switch5/1
  Constant18/1 -> Switch5/3
  Relational Operator3/1 -> Switch4/2
  Constant15/1 -> Switch4/1
  Constant16/1 -> Switch4/3
  Relational Operator2/1 -> Switch3/2
  Constant13/1 -> Switch3/1
  Constant14/1 -> Switch3/3
  Relational Operator1/1 -> Switch1/2
  Constant11/1 -> Switch1/1
  Constant12/1 -> Switch1/3
  Constant10/1 -> Switch2/1
  Logical Operator4/1 -> stError/1
  Constant6/1 -> Switch2/3
  Relational Operator/1 -> Switch2/2
  [status_local] -> Relational Operator7/1
  Constant9/1 -> Relational Operator7/2
  [status_local] -> Relational Operator6/1
  Constant8/1 -> Relational Operator6/2
  [status_local] -> Relational Operator5/1
  Constant7/1 -> Relational Operator5/2
  [status_local] -> Relational Operator4/1
  Constant5/1 -> Relational Operator4/2
  [status_local] -> Relational Operator3/1
  Constant4/1 -> Relational Operator3/2
  [status_local] -> Relational Operator2/1
  Constant3/1 -> Relational Operator2/2
  [status_local] -> Relational Operator1/1
  Constant2/1 -> Relational Operator1/2
  [status_local] -> Relational Operator/1
  status/1 -> [status_local]
  Constant1/1 -> Relational Operator/2

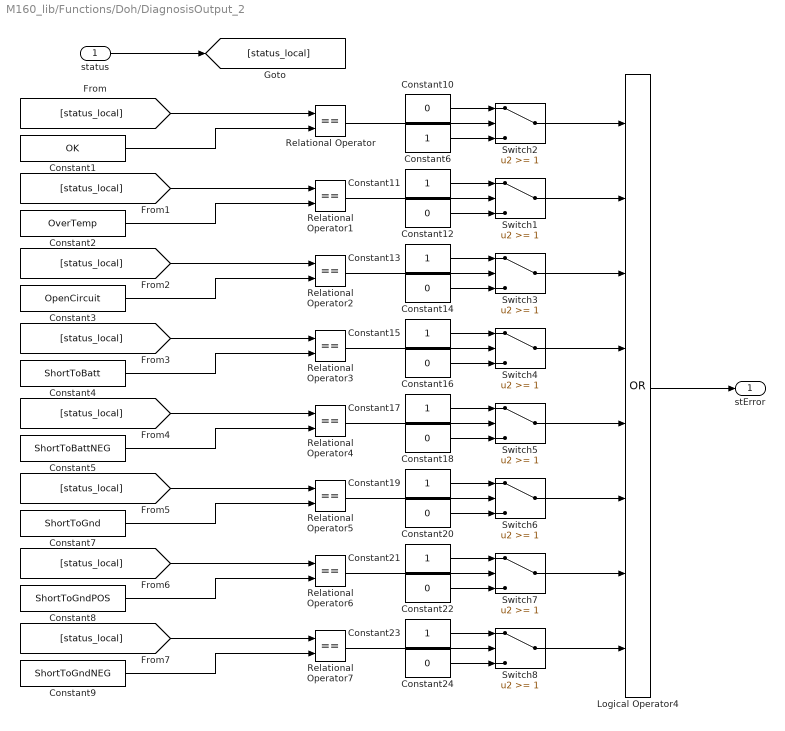
== system M160_lib/Functions/Doh/DiagnosisOutput_2 ==
  status : Inport
  Constant1 : Constant  Value=OK
  Constant{10,12,14,16,18,20,22,24} (8 alike) : Constant  Value=0  OutDataTypeStr=boolean
  Constant{6,11,13,15,17,19,21,23} (8 alike) : Constant  OutDataTypeStr=boolean
  Constant2 : Constant  Value=OverTemp
  Constant3 : Constant  Value=OpenCircuit
  Constant4 : Constant  Value=ShortToBatt
  Constant5 : Constant  Value=ShortToBattNEG
  Constant7 : Constant  Value=ShortToGnd
  Constant8 : Constant  Value=ShortToGndPOS
  Constant9 : Constant  Value=ShortToGndNEG
  Logical Operator4 : Logic  Operator=OR  Inputs=8  AllPortsSameDT=off  OutDataTypeStr=boolean
  Relational Operator{,1..7} (8 alike) : RelationalOperator  Operator===  OutDataTypeStr=boolean
  Switch{1..8} (8 alike) : Switch  Threshold=1
  stError : Outport
  wires:
  Switch8/1 -> Logical Operator4/8
  Switch7/1 -> Logical Operator4/7
  Switch6/1 -> Logical Operator4/6
  Switch5/1 -> Logical Operator4/5
  Switch4/1 -> Logical Operator4/4
  Switch3/1 -> Logical Operator4/3
  Switch1/1 -> Logical Operator4/2
  Switch2/1 -> Logical Operator4/1
  Relational Operator7/1 -> Switch8/2
  Constant23/1 -> Switch8/1
  Constant24/1 -> Switch8/3
  Relational Operator6/1 -> Switch7/2
  Constant21/1 -> Switch7/1
  Constant22/1 -> Switch7/3
  Relational Operator5/1 -> Switch6/2
  Constant19/1 -> Switch6/1
  Constant20/1 -> Switch6/3
  Relational Operator4/1 -> Switch5/2
  Constant17/1 -> Switch5/1
  Constant18/1 -> Switch5/3
  Relational Operator3/1 -> Switch4/2
  Constant15/1 -> Switch4/1
  Constant16/1 -> Switch4/3
  Relational Operator2/1 -> Switch3/2
  Constant13/1 -> Switch3/1
  Constant14/1 -> Switch3/3
  Relational Operator1/1 -> Switch1/2
  Constant11/1 -> Switch1/1
  Constant12/1 -> Switch1/3
  Constant10/1 -> Switch2/1
  Logical Operator4/1 -> stError/1
  Constant6/1 -> Switch2/3
  Relational Operator/1 -> Switch2/2
  [status_local] -> Relational Operator7/1
  Constant9/1 -> Relational Operator7/2
  [status_local] -> Relational Operator6/1
  Constant8/1 -> Relational Operator6/2
  [status_local] -> Relational Operator5/1
  Constant7/1 -> Relational Operator5/2
  [status_local] -> Relational Operator4/1
  Constant5/1 -> Relational Operator4/2
  [status_local] -> Relational Operator3/1
  Constant4/1 -> Relational Operator3/2
  [status_local] -> Relational Operator2/1
  Constant3/1 -> Relational Operator2/2
  [status_local] -> Relational Operator1/1
  Constant2/1 -> Relational Operator1/2
  [status_local] -> Relational Operator/1
  status/1 -> [status_local]
  Constant1/1 -> Relational Operator/2

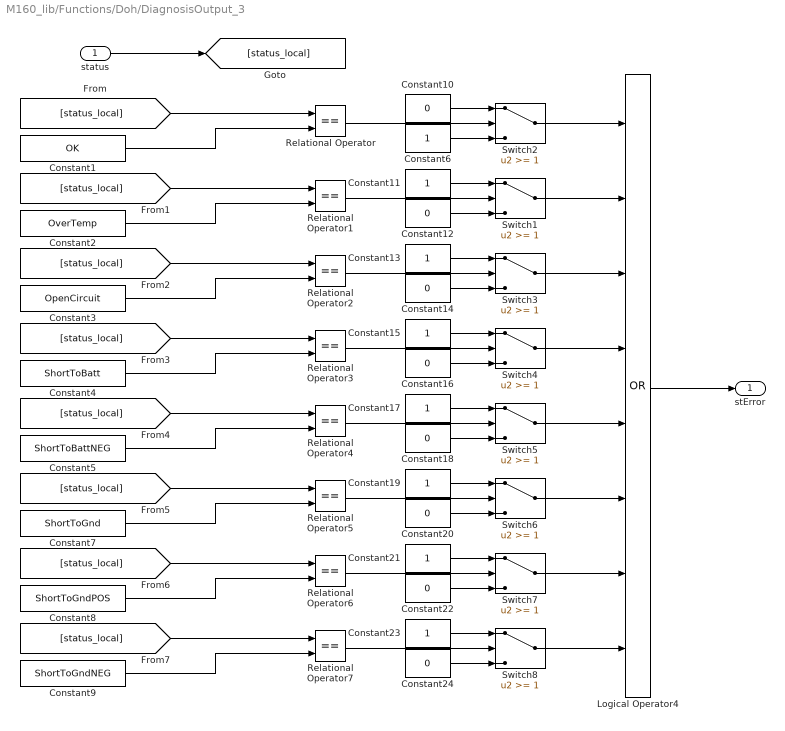
== system M160_lib/Functions/Doh/DiagnosisOutput_3 ==
  status : Inport
  Constant1 : Constant  Value=OK
  Constant{10,12,14,16,18,20,22,24} (8 alike) : Constant  Value=0  OutDataTypeStr=boolean
  Constant{6,11,13,15,17,19,21,23} (8 alike) : Constant  OutDataTypeStr=boolean
  Constant2 : Constant  Value=OverTemp
  Constant3 : Constant  Value=OpenCircuit
  Constant4 : Constant  Value=ShortToBatt
  Constant5 : Constant  Value=ShortToBattNEG
  Constant7 : Constant  Value=ShortToGnd
  Constant8 : Constant  Value=ShortToGndPOS
  Constant9 : Constant  Value=ShortToGndNEG
  Logical Operator4 : Logic  Operator=OR  Inputs=8  AllPortsSameDT=off  OutDataTypeStr=boolean
  Relational Operator{,1..7} (8 alike) : RelationalOperator  Operator===  OutDataTypeStr=boolean
  Switch{1..8} (8 alike) : Switch  Threshold=1
  stError : Outport
  wires:
  Constant1/1 -> Relational Operator/2
  status/1 -> [status_local]
  [status_local] -> Relational Operator/1
  Constant2/1 -> Relational Operator1/2
  [status_local] -> Relational Operator1/1
  Constant3/1 -> Relational Operator2/2
  [status_local] -> Relational Operator2/1
  Constant4/1 -> Relational Operator3/2
  [status_local] -> Relational Operator3/1
  Constant5/1 -> Relational Operator4/2
  [status_local] -> Relational Operator4/1
  Constant7/1 -> Relational Operator5/2
  [status_local] -> Relational Operator5/1
  Constant8/1 -> Relational Operator6/2
  [status_local] -> Relational Operator6/1
  Constant9/1 -> Relational Operator7/2
  [status_local] -> Relational Operator7/1
  Relational Operator/1 -> Switch2/2
  Constant6/1 -> Switch2/3
  Logical Operator4/1 -> stError/1
  Constant10/1 -> Switch2/1
  Constant12/1 -> Switch1/3
  Constant11/1 -> Switch1/1
  Relational Operator1/1 -> Switch1/2
  Constant14/1 -> Switch3/3
  Constant13/1 -> Switch3/1
  Relational Operator2/1 -> Switch3/2
  Constant16/1 -> Switch4/3
  Constant15/1 -> Switch4/1
  Relational Operator3/1 -> Switch4/2
  Constant18/1 -> Switch5/3
  Constant17/1 -> Switch5/1
  Relational Operator4/1 -> Switch5/2
  Constant20/1 -> Switch6/3
  Constant19/1 -> Switch6/1
  Relational Operator5/1 -> Switch6/2
  Constant22/1 -> Switch7/3
  Constant21/1 -> Switch7/1
  Relational Operator6/1 -> Switch7/2
  Constant24/1 -> Switch8/3
  Constant23/1 -> Switch8/1
  Relational Operator7/1 -> Switch8/2
  Switch2/1 -> Logical Operator4/1
  Switch1/1 -> Logical Operator4/2
  Switch3/1 -> Logical Operator4/3
  Switch4/1 -> Logical Operator4/4
  Switch5/1 -> Logical Operator4/5
  Switch6/1 -> Logical Operator4/6
  Switch7/1 -> Logical Operator4/7
  Switch8/1 -> Logical Operator4/8

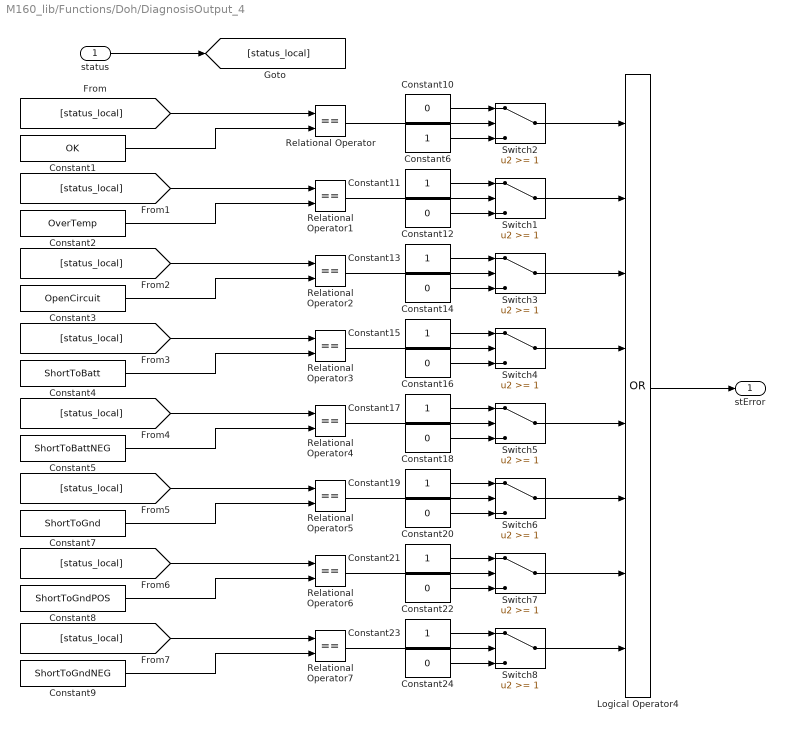
== system M160_lib/Functions/Doh/DiagnosisOutput_4 ==
  status : Inport
  Constant1 : Constant  Value=OK
  Constant{10,12,14,16,18,20,22,24} (8 alike) : Constant  Value=0  OutDataTypeStr=boolean
  Constant{6,11,13,15,17,19,21,23} (8 alike) : Constant  OutDataTypeStr=boolean
  Constant2 : Constant  Value=OverTemp
  Constant3 : Constant  Value=OpenCircuit
  Constant4 : Constant  Value=ShortToBatt
  Constant5 : Constant  Value=ShortToBattNEG
  Constant7 : Constant  Value=ShortToGnd
  Constant8 : Constant  Value=ShortToGndPOS
  Constant9 : Constant  Value=ShortToGndNEG
  Logical Operator4 : Logic  Operator=OR  Inputs=8  AllPortsSameDT=off  OutDataTypeStr=boolean
  Relational Operator{,1..7} (8 alike) : RelationalOperator  Operator===  OutDataTypeStr=boolean
  Switch{1..8} (8 alike) : Switch  Threshold=1
  stError : Outport
  wires:
  Switch8/1 -> Logical Operator4/8
  Switch7/1 -> Logical Operator4/7
  Switch6/1 -> Logical Operator4/6
  Switch5/1 -> Logical Operator4/5
  Switch4/1 -> Logical Operator4/4
  Switch3/1 -> Logical Operator4/3
  Switch1/1 -> Logical Operator4/2
  Switch2/1 -> Logical Operator4/1
  Relational Operator7/1 -> Switch8/2
  Constant23/1 -> Switch8/1
  Constant24/1 -> Switch8/3
  Relational Operator6/1 -> Switch7/2
  Constant21/1 -> Switch7/1
  Constant22/1 -> Switch7/3
  Relational Operator5/1 -> Switch6/2
  Constant19/1 -> Switch6/1
  Constant20/1 -> Switch6/3
  Relational Operator4/1 -> Switch5/2
  Constant17/1 -> Switch5/1
  Constant18/1 -> Switch5/3
  Relational Operator3/1 -> Switch4/2
  Constant15/1 -> Switch4/1
  Constant16/1 -> Switch4/3
  Relational Operator2/1 -> Switch3/2
  Constant13/1 -> Switch3/1
  Constant14/1 -> Switch3/3
  Relational Operator1/1 -> Switch1/2
  Constant11/1 -> Switch1/1
  Constant12/1 -> Switch1/3
  Constant10/1 -> Switch2/1
  Logical Operator4/1 -> stError/1
  Constant6/1 -> Switch2/3
  Relational Operator/1 -> Switch2/2
  [status_local] -> Relational Operator7/1
  Constant9/1 -> Relational Operator7/2
  [status_local] -> Relational Operator6/1
  Constant8/1 -> Relational Operator6/2
  [status_local] -> Relational Operator5/1
  Constant7/1 -> Relational Operator5/2
  [status_local] -> Relational Operator4/1
  Constant5/1 -> Relational Operator4/2
  [status_local] -> Relational Operator3/1
  Constant4/1 -> Relational Operator3/2
  [status_local] -> Relational Operator2/1
  Constant3/1 -> Relational Operator2/2
  [status_local] -> Relational Operator1/1
  Constant2/1 -> Relational Operator1/2
  [status_local] -> Relational Operator/1
  status/1 -> [status_local]
  Constant1/1 -> Relational Operator/2

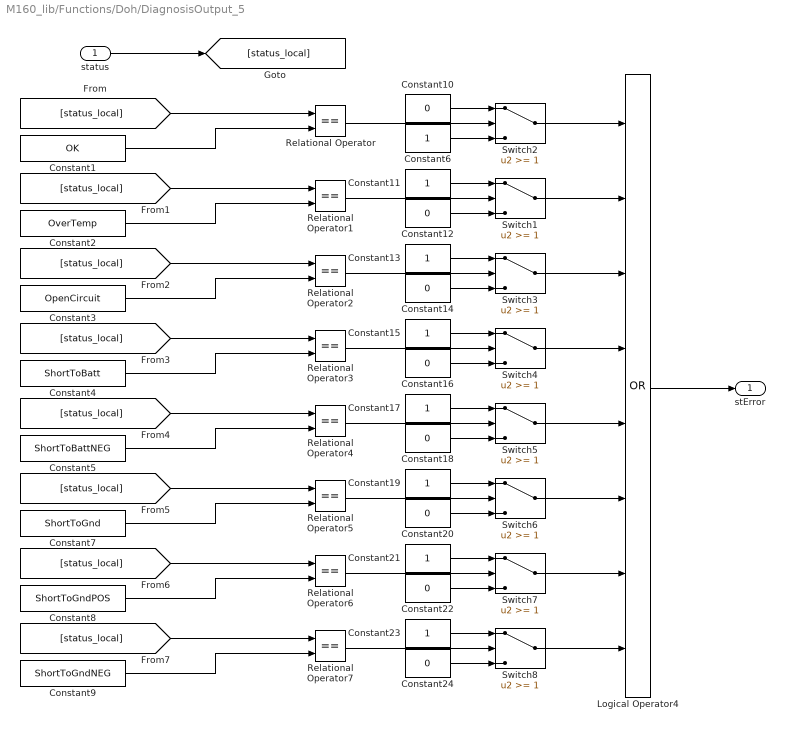
== system M160_lib/Functions/Doh/DiagnosisOutput_5 ==
  status : Inport
  Constant1 : Constant  Value=OK
  Constant{10,12,14,16,18,20,22,24} (8 alike) : Constant  Value=0  OutDataTypeStr=boolean
  Constant{6,11,13,15,17,19,21,23} (8 alike) : Constant  OutDataTypeStr=boolean
  Constant2 : Constant  Value=OverTemp
  Constant3 : Constant  Value=OpenCircuit
  Constant4 : Constant  Value=ShortToBatt
  Constant5 : Constant  Value=ShortToBattNEG
  Constant7 : Constant  Value=ShortToGnd
  Constant8 : Constant  Value=ShortToGndPOS
  Constant9 : Constant  Value=ShortToGndNEG
  Logical Operator4 : Logic  Operator=OR  Inputs=8  AllPortsSameDT=off  OutDataTypeStr=boolean
  Relational Operator{,1..7} (8 alike) : RelationalOperator  Operator===  OutDataTypeStr=boolean
  Switch{1..8} (8 alike) : Switch  Threshold=1
  stError : Outport
  wires:
  Constant1/1 -> Relational Operator/2
  status/1 -> [status_local]
  [status_local] -> Relational Operator/1
  Constant2/1 -> Relational Operator1/2
  [status_local] -> Relational Operator1/1
  Constant3/1 -> Relational Operator2/2
  [status_local] -> Relational Operator2/1
  Constant4/1 -> Relational Operator3/2
  [status_local] -> Relational Operator3/1
  Constant5/1 -> Relational Operator4/2
  [status_local] -> Relational Operator4/1
  Constant7/1 -> Relational Operator5/2
  [status_local] -> Relational Operator5/1
  Constant8/1 -> Relational Operator6/2
  [status_local] -> Relational Operator6/1
  Constant9/1 -> Relational Operator7/2
  [status_local] -> Relational Operator7/1
  Relational Operator/1 -> Switch2/2
  Constant6/1 -> Switch2/3
  Logical Operator4/1 -> stError/1
  Constant10/1 -> Switch2/1
  Constant12/1 -> Switch1/3
  Constant11/1 -> Switch1/1
  Relational Operator1/1 -> Switch1/2
  Constant14/1 -> Switch3/3
  Constant13/1 -> Switch3/1
  Relational Operator2/1 -> Switch3/2
  Constant16/1 -> Switch4/3
  Constant15/1 -> Switch4/1
  Relational Operator3/1 -> Switch4/2
  Constant18/1 -> Switch5/3
  Constant17/1 -> Switch5/1
  Relational Operator4/1 -> Switch5/2
  Constant20/1 -> Switch6/3
  Constant19/1 -> Switch6/1
  Relational Operator5/1 -> Switch6/2
  Constant22/1 -> Switch7/3
  Constant21/1 -> Switch7/1
  Relational Operator6/1 -> Switch7/2
  Constant24/1 -> Switch8/3
  Constant23/1 -> Switch8/1
  Relational Operator7/1 -> Switch8/2
  Switch2/1 -> Logical Operator4/1
  Switch1/1 -> Logical Operator4/2
  Switch3/1 -> Logical Operator4/3
  Switch4/1 -> Logical Operator4/4
  Switch5/1 -> Logical Operator4/5
  Switch6/1 -> Logical Operator4/6
  Switch7/1 -> Logical Operator4/7
  Switch8/1 -> Logical Operator4/8
